simulink library "HeatPump_basic"  (Simulink 8.2)
settings: Solver=ode45  StartTime=0.0  StopTime=10.0  RelTol=1e-3
undefined symbols (not defined in the file): capc, caph, K, UA
libraries: carnot x2
settings Model: Creator=drhf  LastModifiedBy=drhf

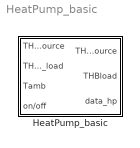
== system HeatPump_basic ==
  HeatPump_basic : Subsystem  mask(heat pump){K=K, caph=caph, capc=capc, UA=UA}
      mask prompts: K "Parameters K (see also HP_param.m)"; caph "thermal capacity hot loop [J/K]"; capc "thermal capacity cold loop [J/K]"; UA "heat loss coefficient [W/K]"
      mask help:
      | Linearized heat pump model, uses measured data according to EN 14511 as input (Schwamberger, K.: Fortschrittsberichete VDI, Nr. 263, 1991).
      | heating power: Qdot_h = K1*Tcold_in + K2*Thot_out + K3
      | electric power: Pel = K4*Tcold_in + K5*Thot_out + K6
      | source power: Qdot_c = -K7*Tcold_in - K8*Thot_out - K9
      | differential equation: cap*dTh/dt = Qdot + mdot*cp*(T_in-T) + UA*(Tamb-T)
      | with: cap = mass * heat_capactiy
      | See hp_param.m for the parameters K1 to K9.
      mask Help: web(fullfile(path_carnot('help'),'HeatPump_basic.html'),'-helpbrowser')
      mask Display: plot(0,-30,120,130,[30,46,36,46,36,46,30],[40,40,50,60,70,80,80],[70,54,64,54,64,54,64,54,64,54,70],[40,40,44,50,55,60,65,70,75,80,80],[56,45],[95,95],[51,51],[82,95])

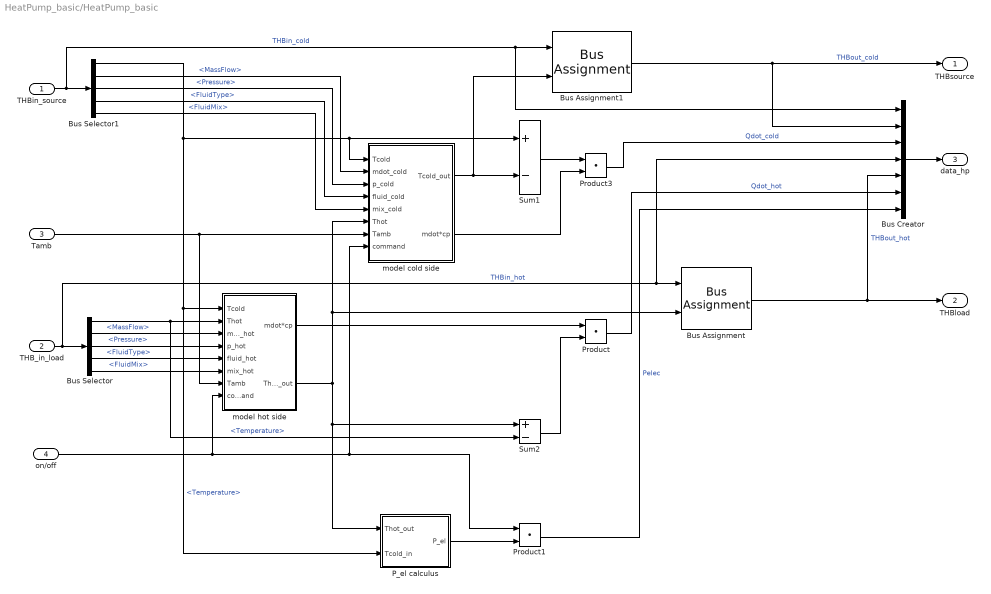
== system HeatPump_basic/HeatPump_basic ==
  THBin_source : Inport
  THB_in_load : Inport  Port=2
  Tamb : Inport  Port=3
  on/off : Inport  Port=4
  Bus Assignment : BusAssignment  AssignedSignals=Temperature
  Bus Assignment1 : BusAssignment  AssignedSignals=Temperature
  Bus Creator : BusCreator  Inputs=7
  Bus Selector : BusSelector  OutputSignals=Temperature,MassFlow,Pressure,FluidType,FluidMix
  Bus Selector1 : BusSelector  OutputSignals=Temperature,MassFlow,Pressure,FluidType,FluidMix
  P_el calculus : Subsystem
  Product : DotProduct  InputSameDT=on  OutDataTypeStr=Inherit: Inherit via internal rule
  Product1 : DotProduct  InputSameDT=on  OutDataTypeStr=Inherit: Inherit via internal rule
  Product3 : DotProduct  InputSameDT=on  OutDataTypeStr=Inherit: Inherit via internal rule
  Sum1 : Sum  Inputs=+-  SaturateOnIntegerOverflow=on  InputSameDT=on  OutDataTypeStr=Inherit: Same as first input
  Sum2 : Sum  Inputs=+-  SaturateOnIntegerOverflow=on  InputSameDT=on  OutDataTypeStr=Inherit: Same as first input
  model cold side : Subsystem
  model hot side : Subsystem
  THBsource : Outport
  THBload : Outport  Port=2
  data_hp : Outport  Port=3
  wires:
  Bus Creator/1 -> data_hp/1
  Bus Assignment1/1 -> Bus Creator/2, THBsource/1  "THBout_cold"
  THBin_source/1 -> Bus Creator/1, Bus Assignment1/1, Bus Selector1/1  "THBin_cold"
  Bus Assignment/1 -> Bus Creator/5, THBload/1  "THBout_hot"
  Tamb/1 -> model hot side/7(Tamb), model cold side/7(Tamb)
  THB_in_load/1 -> Bus Creator/4, Bus Assignment/1, Bus Selector/1  "THBin_hot"
  Bus Selector1/5 -> model cold side/5(mix_cold)  "<FluidMix>"
  Bus Selector1/4 -> model cold side/4(fluid_cold)  "<FluidType>"
  Bus Selector1/3 -> model cold side/3(p_cold)  "<Pressure>"
  Bus Selector/4 -> model hot side/5(fluid_hot)  "<FluidType>"
  Bus Selector/5 -> model hot side/6(mix_hot)  "<FluidMix>"
  Bus Selector/1 -> Sum2/2, model hot side/2(Thot)  "<Temperature>"
  Bus Selector/2 -> model hot side/3(mdot_hot)  "<MassFlow>"
  model hot side/1(mdot*cp) -> Product/1
  Sum2/1 -> Product/2
  Bus Selector1/1 -> P_el calculus/2(Tcold_in), model hot side/1(Tcold), Sum1/1, model cold side/1(Tcold)  "<Temperature>"
  model cold side/1(Tcold_out) -> Sum1/2, Bus Assignment1/2
  Bus Selector/3 -> model hot side/4(p_hot)  "<Pressure>"
  P_el calculus/1(P_el) -> Product1/2
  Product1/1 -> Bus Creator/7  "Pelec"
  model hot side/2(Thot_out) -> Bus Assignment/2, model cold side/6(Thot), P_el calculus/1(Thot_out), Sum2/1
  on/off/1 -> model cold side/8(command), Product1/1, model hot side/8(command)
  Bus Selector1/2 -> model cold side/2(mdot_cold)  "<MassFlow>"
  Sum1/1 -> Product3/1
  model cold side/2(mdot*cp) -> Product3/2
  Product3/1 -> Bus Creator/3  "Qdot_cold"
  Product/1 -> Bus Creator/6  "Qdot_hot"

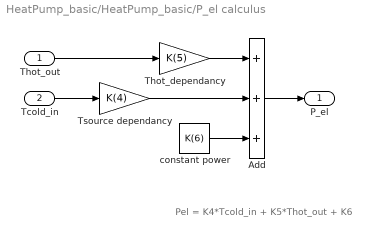
== system HeatPump_basic/HeatPump_basic/P_el calculus ==
  note: Pel = K4*Tcold_in + K5*Thot_out + K6
  Thot_out : Inport
  Tcold_in : Inport  Port=2
  Add : Sum  Inputs=+++
  Thot_dependancy : Gain  Gain=K(5)  SaturateOnIntegerOverflow=on  OutDataTypeStr=Inherit: Same as input  ParamDataTypeStr=Inherit: Same as input
  Tsource dependancy : Gain  Gain=K(4)  SaturateOnIntegerOverflow=on  OutDataTypeStr=Inherit: Same as input  ParamDataTypeStr=Inherit: Same as input
  constant power : Constant  Value=K(6)
  P_el : Outport
  wires:
  constant power/1 -> Add/3
  Tcold_in/1 -> Tsource dependancy/1
  Add/1 -> P_el/1
  Tsource dependancy/1 -> Add/2
  Thot_out/1 -> Thot_dependancy/1
  Thot_dependancy/1 -> Add/1

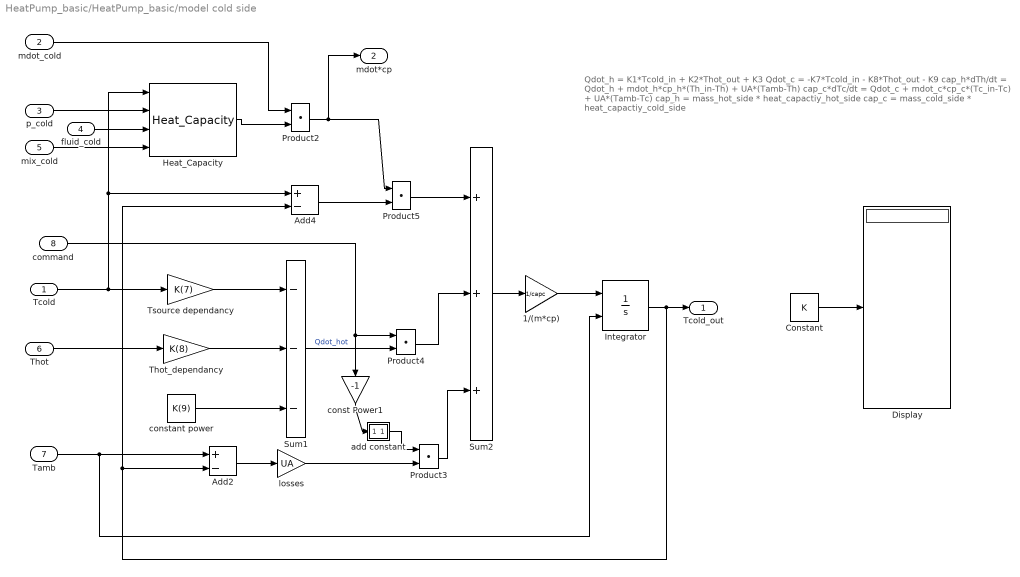
== system HeatPump_basic/HeatPump_basic/model cold side ==
  note: Qdot_h = K1*Tcold_in + K2*Thot_out + K3
      |
      | Qdot_c = -K7*Tcold_in - K8*Thot_out - K9
      |
      | cap_h*dTh/dt = Qdot_h + mdot_h*cp_h*(Th_in-Th) + UA*(Tamb-Th)
      |
      | cap_c*dTc/dt = Qdot_c + mdot_c*cp_c*(Tc_in-Tc) + UA*(Tamb-Tc)
      |
      | cap_h = mass_hot_side * heat_capactiy_hot_side
      |
      | cap_c = mass_cold_side * heat_capactiy_cold_side
  Tcold : Inport
  mdot_cold : Inport  Port=2
  p_cold : Inport  Port=3
  fluid_cold : Inport  Port=4
  mix_cold : Inport  Port=5
  Thot : Inport  Port=6
  Tamb : Inport  Port=7
  command : Inport  Port=8
  1/(m*cp) : Gain  Gain=1/capc
  Add2 : Sum  Inputs=+-
  Add4 : Sum  Inputs=+-
  Constant : Constant  Value=K
  Display : Display
  Heat_Capacity : carnot/Basic/Material_Properties/Heat_Capacity  VariantControl=CarlibClassic  INPUTARGUMENTS=state variables (classic)  DEBUGLEVEL=DEBUGLEVEL  MAXTOTALWARNINGS=inf  MAXCONSECUTIVEWARNINGS=inf  WRITETOFILE=0  FILENAME='errors.txt'
  Integrator : Integrator  InitialConditionSource=external  InitialCondition=25
  Product{2..5} (4 alike) : DotProduct  InputSameDT=on  OutDataTypeStr=Inherit: Inherit via internal rule
  Sum1 : Sum  Inputs=---  SaturateOnIntegerOverflow=on  InputSameDT=on  OutDataTypeStr=Inherit: Same as first input
  Sum2 : Sum  Inputs=3  SaturateOnIntegerOverflow=on  InputSameDT=on  OutDataTypeStr=Inherit: Same as first input
  Thot_dependancy : Gain  Gain=K(8)  SaturateOnIntegerOverflow=on  OutDataTypeStr=Inherit: Same as input  ParamDataTypeStr=Inherit: Same as input
  Tsource dependancy : Gain  Gain=K(7)  SaturateOnIntegerOverflow=on  OutDataTypeStr=Inherit: Same as input  ParamDataTypeStr=Inherit: Same as input
  add constant : Subsystem  mask(add constant){c=+1}
      mask prompts: c "constant c"
      mask help: This block adds a constant c to each element of the input vector.
      mask Help: eval('htmlhelp (''chap_4_2a.htm#add_constant'')')
      mask Display: disp('+c');
  const Power1 : Gain  Gain=-1  SaturateOnIntegerOverflow=on  OutDataTypeStr=Inherit: Same as input  ParamDataTypeStr=Inherit: Same as input
  constant power : Constant  Value=K(9)
  losses : Gain  Gain=UA
  Tcold_out : Outport
  mdot*cp : Outport  Port=2
  wires:
  Integrator/1 -> Add4/2, Add2/2, Tcold_out/1
  Product5/1 -> Sum2/1
  Product4/1 -> Sum2/2
  Product3/1 -> Sum2/3
  Sum2/1 -> 1/(m*cp)/1
  Add4/1 -> Product5/2
  const Power1/1 -> add constant/1(In1)
  add constant/1(Out1) -> Product3/1
  losses/1 -> Product3/2
  command/1 -> const Power1/1, Product4/1
  Tamb/1 -> Integrator/2, Add2/1
  Sum1/1 -> Product4/2  "Qdot_hot"
  constant power/1 -> Sum1/3
  Thot_dependancy/1 -> Sum1/2
  Tsource dependancy/1 -> Sum1/1
  Tcold/1 -> Tsource dependancy/1, Heat_Capacity/1, Add4/1
  Add2/1 -> losses/1
  mdot_cold/1 -> Product2/1
  Heat_Capacity/1 -> Product2/2
  Product2/1 -> Product5/1, mdot*cp/1
  Thot/1 -> Thot_dependancy/1
  p_cold/1 -> Heat_Capacity/2
  mix_cold/1 -> Heat_Capacity/4
  fluid_cold/1 -> Heat_Capacity/3
  1/(m*cp)/1 -> Integrator/1
  Constant/1 -> Display/1

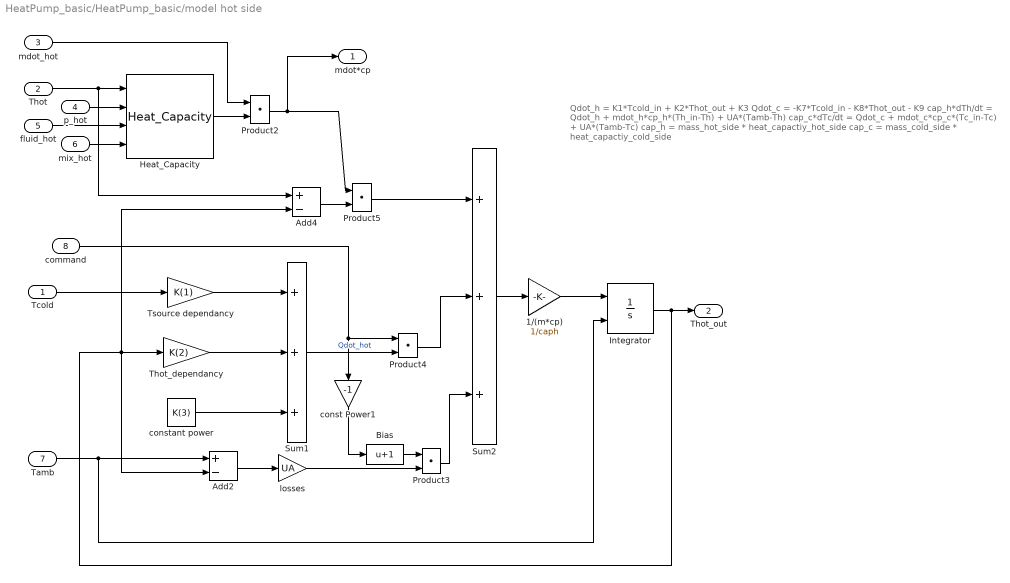
== system HeatPump_basic/HeatPump_basic/model hot side ==
  note: Qdot_h = K1*Tcold_in + K2*Thot_out + K3
      |
      | Qdot_c = -K7*Tcold_in - K8*Thot_out - K9
      |
      | cap_h*dTh/dt = Qdot_h + mdot_h*cp_h*(Th_in-Th) + UA*(Tamb-Th)
      |
      | cap_c*dTc/dt = Qdot_c + mdot_c*cp_c*(Tc_in-Tc) + UA*(Tamb-Tc)
      |
      | cap_h = mass_hot_side * heat_capactiy_hot_side
      |
      | cap_c = mass_cold_side * heat_capactiy_cold_side
  Tcold : Inport
  Thot : Inport  Port=2
  mdot_hot : Inport  Port=3
  p_hot : Inport  Port=4
  fluid_hot : Inport  Port=5
  mix_hot : Inport  Port=6
  Tamb : Inport  Port=7
  command : Inport  Port=8
  1/(m*cp) : Gain  Gain=1/caph
  Add2 : Sum  Inputs=+-
  Add4 : Sum  Inputs=+-
  Bias : Bias  Bias=1
  Heat_Capacity : carnot/Basic/Material_Properties/Heat_Capacity  VariantControl=CarlibClassic  INPUTARGUMENTS=state variables (classic)  DEBUGLEVEL=DEBUGLEVEL  MAXTOTALWARNINGS=inf  MAXCONSECUTIVEWARNINGS=inf  WRITETOFILE=0  FILENAME='errors.txt'
  Integrator : Integrator  InitialConditionSource=external  InitialCondition=25
  Product{2..5} (4 alike) : DotProduct  InputSameDT=on  OutDataTypeStr=Inherit: Inherit via internal rule
  Sum1 : Sum  Inputs=+++  SaturateOnIntegerOverflow=on  InputSameDT=on  OutDataTypeStr=Inherit: Same as first input
  Sum2 : Sum  Inputs=+++  SaturateOnIntegerOverflow=on  InputSameDT=on  OutDataTypeStr=Inherit: Same as first input
  Thot_dependancy : Gain  Gain=K(2)  SaturateOnIntegerOverflow=on  OutDataTypeStr=Inherit: Same as input  ParamDataTypeStr=Inherit: Same as input
  Tsource dependancy : Gain  Gain=K(1)  SaturateOnIntegerOverflow=on  OutDataTypeStr=Inherit: Same as input  ParamDataTypeStr=Inherit: Same as input
  const Power1 : Gain  Gain=-1  SaturateOnIntegerOverflow=on  OutDataTypeStr=Inherit: Same as input  ParamDataTypeStr=Inherit: Same as input
  constant power : Constant  Value=K(3)
  losses : Gain  Gain=UA
  mdot*cp : Outport
  Thot_out : Outport  Port=2
  wires:
  fluid_hot/1 -> Heat_Capacity/3
  mix_hot/1 -> Heat_Capacity/4
  p_hot/1 -> Heat_Capacity/2
  Thot/1 -> Heat_Capacity/1, Add4/1
  Product2/1 -> mdot*cp/1, Product5/1
  Heat_Capacity/1 -> Product2/2
  mdot_hot/1 -> Product2/1
  Add2/1 -> losses/1
  Tcold/1 -> Tsource dependancy/1
  Tsource dependancy/1 -> Sum1/1
  Thot_dependancy/1 -> Sum1/2
  constant power/1 -> Sum1/3
  Sum1/1 -> Product4/2  "Qdot_hot"
  Tamb/1 -> Add2/1, Integrator/2
  command/1 -> Product4/1, const Power1/1
  losses/1 -> Product3/2
  Bias/1 -> Product3/1
  const Power1/1 -> Bias/1
  Add4/1 -> Product5/2
  Sum2/1 -> 1/(m*cp)/1
  1/(m*cp)/1 -> Integrator/1
  Product3/1 -> Sum2/3
  Product4/1 -> Sum2/2
  Product5/1 -> Sum2/1
  Integrator/1 -> Thot_out/1, Add4/2, Thot_dependancy/1, Add2/2

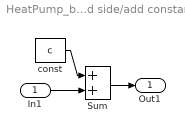
== system HeatPump_basic/HeatPump_basic/model cold side/add constant ==
  In1 : Inport
  Sum : Sum  SaturateOnIntegerOverflow=on  InputSameDT=on  OutDataTypeStr=Inherit: Same as first input
  const : Constant  Value=c
  Out1 : Outport
  wires:
  Sum/1 -> Out1/1
  In1/1 -> Sum/2
  const/1 -> Sum/1
